simulink model "realtime_simu_franka_fr3"  (R2022b)
settings: Solver=FixedStepDiscrete  StartTime=0.0  StopTime=inf  FixedStep=0.001  RelTol=1e-3
PreLoadFcn:
  | set_param(gcs, 'RTWSystemTargetFile', 'franka_emika_panda.tlc');
  | 
  | demos_common_configs();
  | collision_behavior = ones(1,52)*100;
InitFcn:
  | parameters_franka_fr3;
values from neighbouring files (symbols this model uses):
  q_init = [0, -pi/4, 0, -3 * pi/4, 0, pi/2, pi/4]'    [parameters.m]    (also in parameters_franka_fr3.m)
undefined symbols (not defined in the file or in its folder): init_bus_param, MPC12, param_EKF, param_global, param_robot, param_savgol, param_traj, param_vis, v7_kin_int_planner
libraries: franka_simulink_library x5, dspstat3 x2
settings Model: SimulationMode=external  ExtModeTrigDuration=10000  Creator=vasi_ko  LastModifiedBy=rslstudent
settings SolverCC: AlgebraicLoopSolver=TrustRegion
settings DataIOCC: LimitDataPoints=on  SaveFormat=Array  ReturnWorkspaceOutputs=off
settings OptimizationCC: EnhancedBackFolding=on  OptimizeBlockOrder=speed  DifferentSizesBufferReuse=on  OptimizationCustomize=off
settings DebuggingCC: SolverPrmCheckMsg=warning  ParameterTunabilityLossMsg=error  UnconnectedInputMsg=warning  UnconnectedOutputMsg=warning  UnconnectedLineMsg=warning  SFUnexpectedBacktrackingDiag=warning  SFNoUnconditionalDefaultTransitionDiag=warning  SFExecutionAtInitializationDiag=none  SFMachineParentedDataDiag=warning  ArithmeticOperatorsInVariantConditions=warning
settings HardwareCC: ProdBitPerLong=64  ProdHWDeviceType=Intel->x86-64 (Linux 64)
settings ModelReferenceCC: UpdateModelReferenceTargets=IfOutOfDate  EnableRefExpFcnMdlSchedulingChecks=on  PropagateSignalLabelsOutOfModel=off
settings SFSimCC: SimUseLocalCustomCode=off  MATLABDynamicMemAlloc=off  CustomCodeUndefinedFunction=UseInterfaceOnly  SimTargetLang=C++
settings RTWCC: SystemTargetFile=franka_emika_panda.tlc  RTWUseLocalCustomCode=off  Toolchain=Franka Simulink | gmake (64-bit linux)  BuildConfiguration=Faster Runs  TargetLang=C++
settings CodeAppCC: OperatorAnnotations=on
settings STFCustomTargetCC: TargetLangStandard=C99 (ISO)  ModelReferenceCompliant=off  CombineOutputUpdateFcns=on  MatFileLogging=on  UseToolchainInfoCompliant=on  SystemTargetFile=franka_emika_panda.tlc
settings GRTTargetCC: ModelReferenceCompliant=off  ParMdlRefBuildCompliant=off  CompOptLevelCompliant=off  ConcurrentExecutionCompliant=off  CPPClassGenCompliant=off  ExtModeStaticAlloc=on  ExtModeTransport=1  ExtModeMexFile=ext_xcp  ExtModeIntrfLevel=Level2 - Open
settings ConfigComp: CovMetricSettings=dw  CovSaveCumulativeToWorkspaceVar=on  CovSaveSingleToWorkspaceVar=on  CovExternalEMLEnable=off  CovSFcnEnable=off

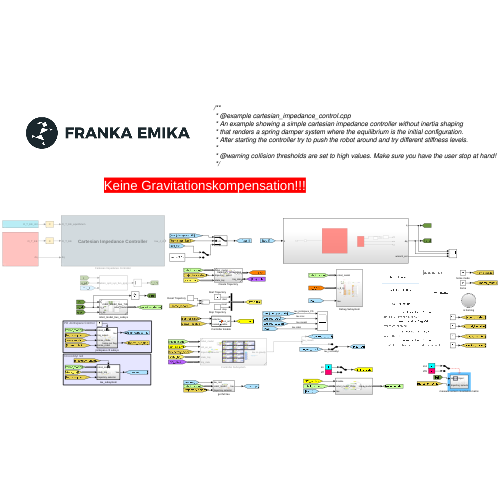
[thumbnail: Simulink's stored preview of the top-level diagram]
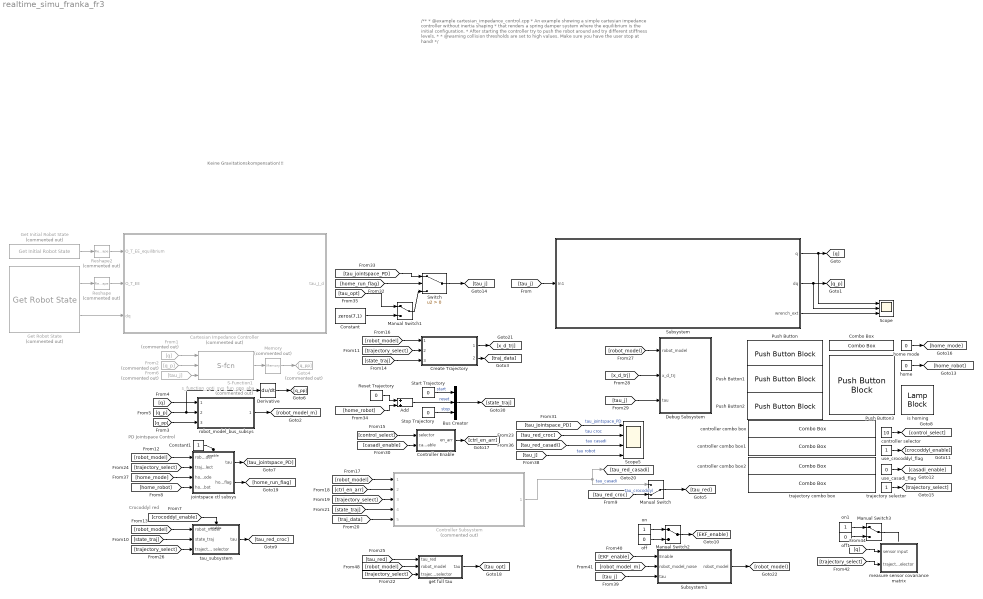
== system realtime_simu_franka_fr3 ==
  note: Crocoddyl red
  note: PD Jointspace Control
  note: Keine Gravitationskompensation!!!
  note: /**
      |  * @example cartesian_impedance_control.cpp
      |  * An example showing a simple cartesian impedance controller without inertia shaping
      |  * that renders a spring damper system where the equilibrium is the initial configuration.
      |  * After starting the controller try to push the robot around and try different stiffness levels.
      |  *
      |  * @warning collision thresholds are set to high values. Make sure you have the user stop at hand!
      |  */
  Add : Sum
  Bus Creator : BusCreator  Inputs=3  OutDataTypeStr=Bus: state_traj_bus
      settings: InheritFromInputs=off
  Cartesian Impedance Controller : Subsystem  Commented=on
      mask Display:
      | disp('{\bf\fontsize{18}Cartesian Impedance Controller}', 'texmode','on');
      | 
      | block_icon('Controller')
      | 
      | port_label('output',1,'tau_J_d');
      | 
      | port_label('input',1,'O_T_EE_equilibrium');
      | port_label('input',2,'O_T_EE');
      | port_label('input',3,'dq');
  Combo Box : ComboBox  LabelPosition=Hide  SelectedLabel=Home init pose
      settings: Values={{'Home init pose', 'Trajectory init pose'}, [0 1]}
  Constant : Constant  Value=zeros(7,1)
  Constant1 : Constant
  Controller Enable : MATLAB Function  TreatAsAtomicUnit=on
  Controller Subsystem : Subsystem  Commented=on  ReferencedSubsystem=controller_ref_subsys
  Create Trajectory : Subsystem  ReferencedSubsystem=trajectory_generation_ref_subsys_7dof
  Debug Subsystem : Subsystem
  Derivative : Derivative
  From1 : From  Commented=on  GotoTag=q
  From2 : From  Commented=on  GotoTag=q_p
  From6 : From  Commented=on  GotoTag=tau_j
  Get Initial Robot State : franka_simulink_library/Get Initial Robot State  Commented=on  robot_ip=robot_ip  signals_requested='O_T_EE'
      settings: SourceProductName=Franka Emika Simulink Support Package
  Get Robot State : franka_simulink_library/Get Robot State  Commented=on  robot_ip=robot_ip  signals_requested='O_T_EE dq'
      settings: SourceProductName=Franka Emika Simulink Support Package
  Goto4 : Goto  Commented=on  GotoTag=q_pp
  Manual Switch : ManualSwitch  CurrentSetting=0
  Manual Switch1 : ManualSwitch
  Manual Switch2 : ManualSwitch
  Manual Switch3 : ManualSwitch
  Memory : Memory  Commented=on  InitialCondition=zeros(7,1)
  Push Button : PushButtonBlock  ButtonText=Start Trajectory  OffValue=0.000000
  Push Button1 : PushButtonBlock  ButtonText=Reset Trajectory  OffValue=0.000000
  Push Button2 : PushButtonBlock  ButtonText=Stop Trajectory  OffValue=0.000000
  Push Button3 : PushButtonBlock  ButtonText=HOME ROBOT  OffValue=0.000000
  Reset Trajectory : Constant  Value=0
  Reshape : Reshape  Commented=on  OutputDimensionality=Customize  OutputDimensions=[4,4]
  Reshape2 : Reshape  Commented=on  OutputDimensionality=Customize  OutputDimensions=[4,4]
  S-Function1 : S-Function  Commented=on  FunctionName=s_function_opti_sys_fun_qpp_aba  SFunctionModules='sys_fun_qpp_aba'  SFunctionDeploymentMode=off  EnableBusSupport=off
  Scope : Scope  NumInputPorts=3
  Scope5 : Scope  NumInputPorts=4
  Start Trajectory : Constant  Value=0
  Stop Trajectory : Constant  Value=0
  Subsystem : Subsystem
  Subsystem1 : Subsystem
  Switch : Switch  Criteria=u2 > Threshold  SaturateOnIntegerOverflow=off  InputSameDT=off
  controller combo box : ComboBox  SelectedLabel=MPC12 (v7_kin_int_planner)
      settings: Values={{'Cartesian CT Control', 'Cartesian PD+ Control', 'MPC01', 'MPC6 (v3_quat)', 'MPC7 (v3_rpy)', 'MPC8 (v4_kin_int)', 'MPC9 (v4_kin_int_refsys)', 'MPC10 (v5_kin_dev)', 'MPC11 (v6_kin_int_pathfollow)', 'MPC12 (v7_kin_int_planner)', 'MPC13 (v8_kin_dev_planner)'}, [1 2 3 4 5 6 7 8 9 10 11]}
  controller combo box1 : ComboBox  SelectedLabel=Croccodyl Enabled
      settings: Values={{'Croccodyl Enabled', 'Croccodyl Disabled'}, [1 0]}
  controller combo box2 : ComboBox  SelectedLabel=Casadi Disabled
      settings: Values={{'Casadi Enabled', 'Casadi Disabled'}, [1 0]}
  controller selector : Constant  Value=10  OutDataTypeStr=uint32  SampleTime=-1
  get full tau : Subsystem
  home : Constant  Value=0
  home mode : Constant  Value=0
  is homing : LampBlock  LabelPosition=Hide
  jointspace ctl subsys : Subsystem
  measure sensor covariance matrix : Subsystem
  off : Constant  Value=0
  off1 : Constant  Value=0
  on : Constant
  on1 : Constant
  robot_model_bus_subsys : Subsystem  ReferencedSubsystem=robot_model_bus_7dof_ref_subsys
  tau_subsystem : Subsystem
  trajectory combo box : ComboBox  SelectedLabel=1: Singularity stretched arm out, Polynomial, Workspace
      settings: Values={{'1: Singularity stretched arm out, Polynomial, Workspace', '2: Singularity stretched arm in, Polynomial, Workspace', '3: Wrist singularity 1, Polynomial, Workspace', '4: Wrist singularity 1, Polynomial, Jointspace', '5: Shoulder - Wrist singularity 1, Polynomial, Workspace'}, [1 2 3 4 5]}
  trajectory selector : Constant  OutDataTypeStr=uint32  SampleTime=-1
  use_casadi_flag : Constant  Value=0
  use_crocoddyl_flag : Constant
  wires:
  Reshape2/1 -> Cartesian Impedance Controller/1(O_T_EE_equilibrium)
  Get Initial Robot State/1 -> Reshape2/1
  Subsystem/1(q) -> Scope/1, [q]
  Subsystem/2(dq) -> Scope/2, [q_p]
  Get Robot State/2 -> Cartesian Impedance Controller/3(dq)
  Reshape/1 -> Cartesian Impedance Controller/2(O_T_EE)
  Get Robot State/1 -> Reshape/1
  Subsystem/3(wrench_ext) -> Scope/3
  [tau_jointspace_PD] -> Scope5/1  "tau_jointspace_PD"
  [tau_j] -> Subsystem/1(In1)
  [q] -> robot_model_bus_subsys/1
  robot_model_bus_subsys/1 -> [robot_model_m]
  [q_p] -> Derivative/1, robot_model_bus_subsys/2
  [q_pp] -> robot_model_bus_subsys/3
  From6/1 -> S-Function1/3
  From1/1 -> S-Function1/1
  From2/1 -> S-Function1/2
  Start Trajectory/1 -> Bus Creator/1  "start"
  Stop Trajectory/1 -> Bus Creator/3  "stop"
  Bus Creator/1 -> [state_traj]
  Constant1/1 -> jointspace ctl subsys/Enable
  [robot_model] -> jointspace ctl subsys/1(robot_model)
  jointspace ctl subsys/1(tau) -> [tau_jointspace_PD]
  [robot_model] -> tau_subsystem/1(robot_model)
  tau_subsystem/1(tau) -> [tau_red_croc]
  [control_select] -> Controller Enable/1(selector)
  Controller Enable/1(en_arr) -> [ctrl_en_arr]
  [robot_model] -> Controller Subsystem/1
  [ctrl_en_arr] -> Controller Subsystem/2
  [trajectory_select] -> Controller Subsystem/3
  [tau_red_croc] -> Manual Switch/2  "tau_crocoddyl"
  [state_traj] -> tau_subsystem/2(state_traj)
  [trajectory_select] -> get full tau/3(trajectory selector)
  [robot_model] -> get full tau/2(robot_model)
  [tau_red] -> get full tau/1(tau_red)
  get full tau/1(tau) -> [tau_opt]
  Manual Switch/1 -> [tau_red]
  Controller Subsystem/1 -> Manual Switch/1, [tau_red_casadi]  "tau_casadi"
  [trajectory_select] -> tau_subsystem/3(trajectory selector)
  [tau_red_croc] -> Scope5/2  "tau croc"
  [crocoddyl_enable] -> tau_subsystem/Enable
  [robot_model] -> Debug Subsystem/1(robot_model)
  [x_d_trj] -> Debug Subsystem/2(x_d_trj)
  [tau_j] -> Debug Subsystem/3(tau)
  Derivative/1 -> [q_pp]
  use_crocoddyl_flag/1 -> [crocoddyl_enable]
  use_casadi_flag/1 -> [casadi_enable]
  [casadi_enable] -> Controller Enable/2(casadi_enable)
  S-Function1/1 -> Memory/1
  Memory/1 -> Goto4/1
  home/1 -> [home_robot]
  [home_robot] -> jointspace ctl subsys/4(home_robot)
  jointspace ctl subsys/2(home run flag) -> [home_run_flag]
  [home_run_flag] -> Switch/2
  [tau_jointspace_PD] -> Switch/1
  Reset Trajectory/1 -> Add/1
  Add/1 -> Bus Creator/2  "reset"
  [home_robot] -> Add/2
  [tau_red_casadi] -> Scope5/3  "tau casadi"
  Create Trajectory/2 -> [traj_data]
  [robot_model] -> Create Trajectory/1
  [trajectory_select] -> Create Trajectory/2
  Create Trajectory/1 -> [x_d_trj]
  [state_traj] -> Create Trajectory/3
  controller selector/1 -> [control_select]
  trajectory selector/1 -> [trajectory_select]
  home mode/1 -> [home_mode]
  [home_mode] -> jointspace ctl subsys/3(home_mode)
  [trajectory_select] -> jointspace ctl subsys/2(traj_select)
  [state_traj] -> Controller Subsystem/4
  [traj_data] -> Controller Subsystem/5
  [tau_j] -> Scope5/4  "tau robot"
  Constant/1 -> Manual Switch1/2
  [tau_opt] -> Manual Switch1/1
  Manual Switch1/1 -> Switch/3
  Switch/1 -> [tau_j]
  on/1 -> Manual Switch2/1
  Manual Switch2/1 -> [EKF_enable]
  [robot_model_m] -> Subsystem1/2(robot_model_noise)
  [tau_j] -> Subsystem1/3(tau)
  off/1 -> Manual Switch2/2
  [EKF_enable] -> Subsystem1/1(Enable)
  Subsystem1/1(robot_model) -> [robot_model]
  [q] -> measure sensor covariance matrix/1(sensor input)
  off1/1 -> Manual Switch3/2
  on1/1 -> Manual Switch3/1
  Manual Switch3/1 -> ?
  [trajectory_select] -> measure sensor covariance matrix/2(trajectory selector)

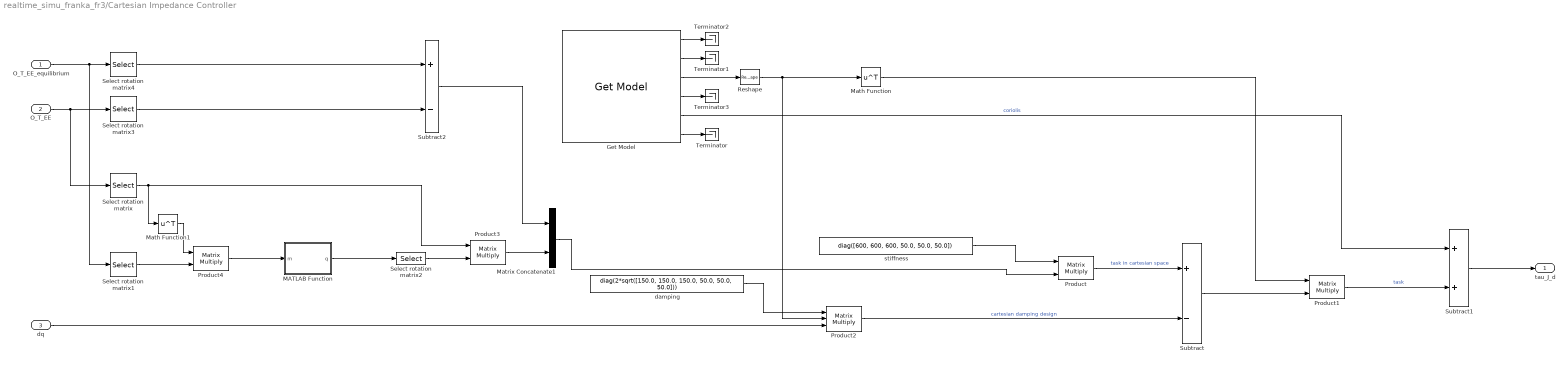
== system realtime_simu_franka_fr3/Cartesian Impedance Controller ==
  O_T_EE_equilibrium : Inport
  O_T_EE : Inport  Port=2
  dq : Inport  Port=3
  Get Model : franka_simulink_library/Get Model  robot_ip=robot_ip
      settings: SourceProductName=Franka Emika Simulink Support Package
  MATLAB Function : MATLAB Function  TreatAsAtomicUnit=on
  Math Function : Math  Operator=transpose  SignedPower=on
  Math Function1 : Math  Operator=transpose  SignedPower=on
  Matrix Concatenate1 : Concatenate
  Product{,1,3..4} (4 alike) : Product  Multiplication=Matrix(*)
  Product2 : Product  Inputs=3  Multiplication=Matrix(*)
  Reshape : Reshape  OutputDimensionality=Customize  OutputDimensions=[6,7]
  Select rotation matrix : Selector  NumberOfDimensions=2  InputPortWidth=3  IndexOptions=Index vector (dialog),Index vector (dialog)  Indices=[1,2,3],[1 2 3]  OutputSizes=1
  Select rotation matrix1 : Selector  NumberOfDimensions=2  InputPortWidth=3  IndexOptions=Index vector (dialog),Index vector (dialog)  Indices=[1,2,3],[1 2 3]  OutputSizes=1
  Select rotation matrix2 : Selector  InputPortWidth=4  IndexOptions=Index vector (dialog)  Indices=[2,3,4]  OutputSizes=1
  Select rotation matrix3 : Selector  NumberOfDimensions=2  InputPortWidth=3  IndexOptions=Index vector (dialog),Index vector (dialog)  Indices=[1,2,3],[4]  OutputSizes=1
  Select rotation matrix4 : Selector  NumberOfDimensions=2  InputPortWidth=3  IndexOptions=Index vector (dialog),Index vector (dialog)  Indices=[1,2,3],[4]  OutputSizes=1
  Subtract : Sum  Inputs=+-
  Subtract1 : Sum
  Subtract2 : Sum  Inputs=+-
  Terminator{,1..3} (4 alike) : Terminator
  damping : Constant  Value=diag(2*sqrt([150.0, 150.0, 150.0, 50.0, 50.0, 50.0]))  VectorParams1D=off
  stiffness : Constant  Value=diag([600, 600, 600, 50.0, 50.0, 50.0])  VectorParams1D=off
  tau_J_d : Outport  VectorParamsAs1DForOutWhenUnconnected=off
  wires:
  Get Model/6 -> Terminator/1
  Get Model/2 -> Terminator1/1
  Get Model/1 -> Terminator2/1
  Get Model/4 -> Terminator3/1
  Get Model/3 -> Reshape/1
  Reshape/1 -> Product2/2, Math Function/1
  stiffness/1 -> Product/1
  Math Function/1 -> Product1/1
  Product/1 -> Subtract/1  "task in cartesian space"
  Product2/1 -> Subtract/2  "cartesian damping design"
  Get Model/5 -> Subtract1/1  "coriolis"
  dq/1 -> Product2/3
  damping/1 -> Product2/1
  Subtract1/1 -> tau_J_d/1
  Product1/1 -> Subtract1/2  "task"
  O_T_EE/1 -> Select rotation matrix3/1, Select rotation matrix/1
  O_T_EE_equilibrium/1 -> Select rotation matrix4/1, Select rotation matrix1/1
  Select rotation matrix4/1 -> Subtract2/1
  Select rotation matrix3/1 -> Subtract2/2
  Subtract2/1 -> Matrix Concatenate1/1
  MATLAB Function/1(q) -> Select rotation matrix2/1
  Product4/1 -> MATLAB Function/1(m)
  Subtract/1 -> Product1/2
  Select rotation matrix2/1 -> Product3/2
  Matrix Concatenate1/1 -> Product/2
  Select rotation matrix/1 -> Math Function1/1, Product3/1
  Product3/1 -> Matrix Concatenate1/2
  Select rotation matrix1/1 -> Product4/2
  Math Function1/1 -> Product4/1

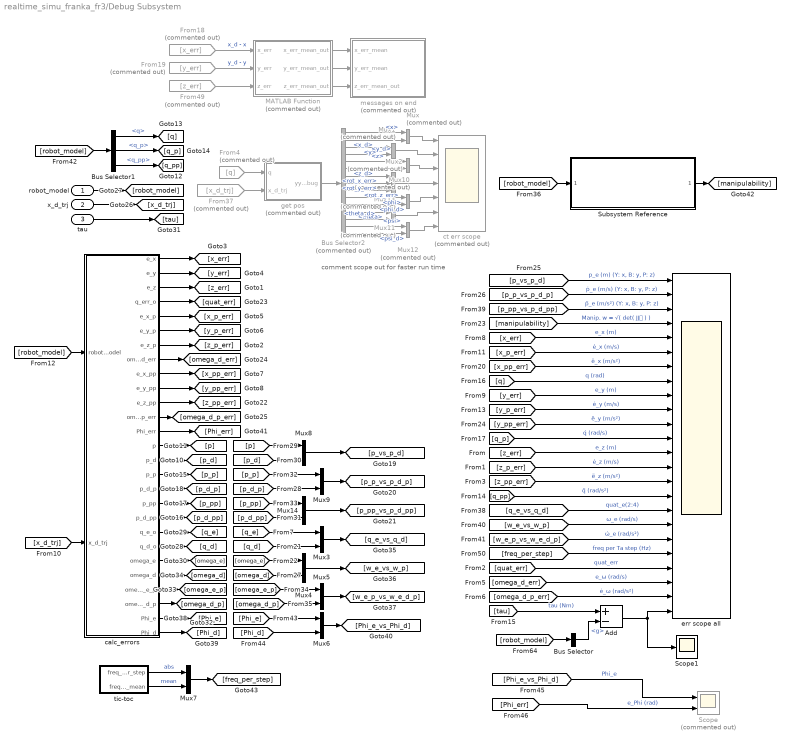
== system realtime_simu_franka_fr3/Debug Subsystem ==
  note: comment scope out for faster run time
  robot_model : Inport
  x_d_trj : Inport  Port=2
  tau : Inport  Port=3
  Add : Sum  Inputs=+-
  Bus Selector : BusSelector  OutputSignals=g
  Bus Selector1 : BusSelector  OutputSignals=q,q_p,q_pp
  Bus Selector2 : BusSelector  Commented=on  OutputSignals=x,x_d,y,y_d,z,z_d,rot_x_err,rot_y_err,rot_z_err,phi,phi_d,theta,theta_d,psi,psi_d
  From18 : From  Commented=on  GotoTag=x_err
  From19 : From  Commented=on  GotoTag=y_err
  From37 : From  Commented=on  GotoTag=x_d_trj
  From4 : From  Commented=on  GotoTag=q
  From49 : From  Commented=on  GotoTag=z_err
  MATLAB Function : MATLAB Function  Commented=on  TreatAsAtomicUnit=on
  Mux{,1..2,10..12} (6 alike) : Mux  Commented=on  Inputs=2
  Mux13 : Mux  Commented=on  Inputs=3
  Mux{3..9,14} (8 alike) : Mux  Inputs=2
  Scope : Scope  Commented=on  NumInputPorts=2
  Scope1 : Scope
  Subsystem Reference : Subsystem  ReferencedSubsystem=manipulability_and_collinearity
  calc_errors : MATLAB Function  TreatAsAtomicUnit=on
  ct err scope : Scope  Commented=on  NumInputPorts=7
  err scope all : Scope  NumInputPorts=24
  get pos : MATLAB Function  Commented=on  TreatAsAtomicUnit=on  SystemSampleTime=param_global.Ta
  messages on end : Subsystem  Commented=on
  tic-toc : Subsystem
  wires:
  Bus Selector1/1 -> [q]  "<q>"
  Bus Selector1/2 -> [q_p]  "<q_p>"
  Bus Selector1/3 -> [q_pp]  "<q_pp>"
  From4/1 -> get pos/1(q)
  x_d_trj/1 -> [x_d_trj]
  robot_model/1 -> [robot_model]
  tau/1 -> [tau]
  From37/1 -> get pos/2(x_d_trj)
  get pos/1(yy_debug) -> Bus Selector2/1
  Mux/1 -> ct err scope/1
  Mux1/1 -> ct err scope/2
  Mux2/1 -> ct err scope/3
  Mux10/1 -> ct err scope/5
  Mux11/1 -> ct err scope/6
  Mux12/1 -> ct err scope/7
  Mux13/1 -> ct err scope/4
  Bus Selector2/1 -> Mux/1  "<x>"
  Bus Selector2/2 -> Mux/2  "<x_d>"
  Bus Selector2/3 -> Mux1/1  "<y>"
  Bus Selector2/4 -> Mux1/2  "<y_d>"
  Bus Selector2/5 -> Mux2/1  "<z>"
  Bus Selector2/6 -> Mux2/2  "<z_d>"
  Bus Selector2/7 -> Mux13/1  "<rot_x_err>"
  Bus Selector2/8 -> Mux13/2  "<rot_y_err>"
  Bus Selector2/9 -> Mux13/3  "<rot_z_err>"
  Bus Selector2/10 -> Mux10/1  "<phi>"
  Bus Selector2/11 -> Mux10/2  "<phi_d>"
  Bus Selector2/12 -> Mux11/1  "<theta>"
  Bus Selector2/13 -> Mux11/2  "<theta_d>"
  Bus Selector2/14 -> Mux12/1  "<psi>"
  Bus Selector2/15 -> Mux12/2  "<psi_d>"
  From18/1 -> MATLAB Function/1(x_err)  "x_d - x"
  From19/1 -> MATLAB Function/2(y_err)  "y_d - y"
  MATLAB Function/2(y_err_mean_out) -> messages on end/2(y_err_mean)
  MATLAB Function/1(x_err_mean_out) -> messages on end/1(x_err_mean)
  [robot_model] -> calc_errors/1(robot_model)
  [x_d_trj] -> calc_errors/2(x_d_trj)
  calc_errors/1(e_x) -> [x_err]
  calc_errors/2(e_y) -> [y_err]
  calc_errors/5(e_x_p) -> [x_p_err]
  calc_errors/6(e_y_p) -> [y_p_err]
  calc_errors/9(e_x_pp) -> [x_pp_err]
  calc_errors/10(e_y_pp) -> [y_pp_err]
  [manipulability] -> err scope all/4  "Manip. w = √( det( JJ⸆ ) )"
  [x_err] -> err scope all/5  "e_x (m)"
  [y_err] -> err scope all/9  "e_y (m)"
  [x_p_err] -> err scope all/6  "ė_x (m/s)"
  [y_p_err] -> err scope all/10  "ė_y (m/s)"
  [x_pp_err] -> err scope all/7  "ё_x (m/s²)"
  [y_pp_err] -> err scope all/11  "ё_y (m/s²)"
  [q] -> err scope all/8  "q (rad)"
  [q_p] -> err scope all/12  "q̇ (rad/s)"
  [q_pp] -> err scope all/16  "q̈ (rad/s²)"
  [p_d_p] -> Mux9/2
  [p_p] -> Mux9/1
  [p_d] -> Mux8/2
  [p] -> Mux8/1
  [p_pp] -> Mux14/1
  [p_d_pp] -> Mux14/2
  [p_p_vs_p_d_p] -> err scope all/2  "ṗ_e (m/s) (Y: x, B: y, P: z)"
  [p_vs_p_d] -> err scope all/1  "p_e (m) (Y: x, B: y, P: z)"
  [p_pp_vs_p_d_pp] -> err scope all/3  "p̈_e (m/s²) (Y: x, B: y, P: z)"
  Mux8/1 -> [p_vs_p_d]
  Mux9/1 -> [p_p_vs_p_d_p]
  Mux14/1 -> [p_pp_vs_p_d_pp]
  calc_errors/14(p) -> [p]
  calc_errors/15(p_d) -> [p_d]
  calc_errors/16(p_p) -> [p_p]
  calc_errors/17(p_d_p) -> [p_d_p]
  calc_errors/18(p_pp) -> [p_pp]
  calc_errors/19(p_d_pp) -> [p_d_pp]
  calc_errors/3(e_z) -> [z_err]
  calc_errors/7(e_z_p) -> [z_p_err]
  calc_errors/11(e_z_pp) -> [z_pp_err]
  [z_err] -> err scope all/13  "e_z (m)"
  [z_p_err] -> err scope all/14  "ė_z (m/s)"
  [z_pp_err] -> err scope all/15  "ё_z (m/s²)"
  calc_errors/4(q_err_o) -> [quat_err]
  calc_errors/12(omega_d_p_err) -> [omega_d_p_err]
  calc_errors/8(omega_d_err) -> [omega_d_err]
  [quat_err] -> err scope all/21  "quat_err"
  [omega_d_err] -> err scope all/22  "e_ω (rad/s)"
  [omega_d_p_err] -> err scope all/23  "ė_ω (rad/s²)"
  calc_errors/20(q_e_o) -> [q_e]
  calc_errors/21(q_d_o) -> [q_d]
  calc_errors/22(omega_e) -> [omega_e]
  calc_errors/23(omega_d) -> [omega_d]
  calc_errors/24(omega_e_p) -> [omega_e_p]
  calc_errors/25(omega_d_p) -> [omega_d_p]
  [q_e] -> Mux3/1
  [q_d] -> Mux3/2
  [omega_e] -> Mux4/1
  [omega_d] -> Mux4/2
  [omega_e_p] -> Mux5/1
  [omega_d_p] -> Mux5/2
  Mux3/1 -> [q_e_vs_q_d]
  Mux4/1 -> [w_e_vs_w_p]
  Mux5/1 -> [w_e_p_vs_w_e_d_p]
  [q_e_vs_q_d] -> err scope all/17  "quat_e(2:4)"
  [w_e_vs_w_p] -> err scope all/18  "ω_e (rad/s)"
  [w_e_p_vs_w_e_d_p] -> err scope all/19  "ὠ_e (rad/s²)"
  calc_errors/26(Phi_e) -> [Phi_e]
  calc_errors/27(Phi_d) -> [Phi_d]
  [Phi_d] -> Mux6/2
  [Phi_e] -> Mux6/1
  Mux6/1 -> [Phi_e_vs_Phi_d]
  [Phi_e_vs_Phi_d] -> Scope/1  "Phi_e"
  calc_errors/13(Phi_err) -> [Phi_err]
  [Phi_err] -> Scope/2  "e_Phi (rad)"
  From49/1 -> MATLAB Function/3(z_err)
  MATLAB Function/3(z_err_mean_out) -> messages on end/3(z_err_mean_out)
  [freq_per_step] -> err scope all/20  "freq per Ta step (Hz)"
  Subsystem Reference/1 -> [manipulability]
  [robot_model] -> Subsystem Reference/1
  Mux7/1 -> [freq_per_step]
  tic-toc/1(freq_per_step) -> Mux7/1  "abs"
  tic-toc/2(freq_per_step_mean) -> Mux7/2  "mean"
  [robot_model] -> Bus Selector/1
  [tau] -> Add/1  "tau (Nm)"
  Add/1 -> err scope all/24, Scope1/1
  Bus Selector/1 -> Add/2  "<g>"
  [robot_model] -> Bus Selector1/1

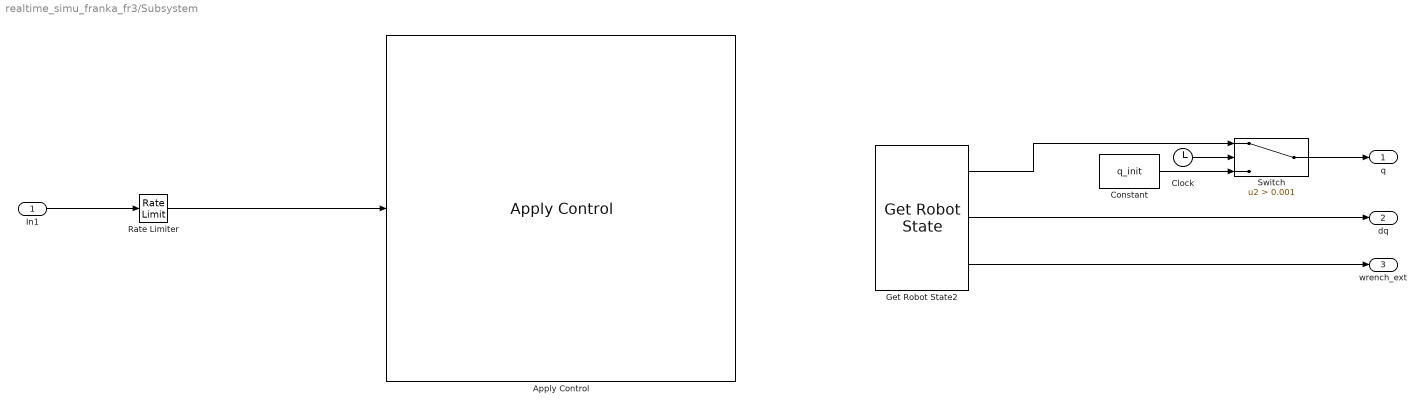
== system realtime_simu_franka_fr3/Subsystem ==
  In1 : Inport
  Apply Control : franka_simulink_library/Apply Control  robot_ip=robot_ip  gripper_attached=off  control_mode=Torque Control  controller_choice=Joint Impedance Controller  elbow_control=on  collision_thresholds=100*ones(1,52)  joint_impedance=joint_impedance  cartesian_impedance=cartesian_impedance  load_inertia=load_inertia  EE_T_K=EE_T_K  init_joint_configuration_req=on  init_joint_configuration=q_init'
      settings: SourceProductName=Franka Emika Simulink Support Package
  Clock : Clock
  Constant : Constant  Value=q_init
  Get Robot State2 : franka_simulink_library/Get Robot State  robot_ip=robot_ip  signals_requested='q dq O_F_ext_hat_K'
      settings: SourceProductName=Franka Emika Simulink Support Package
  Rate Limiter : RateLimiter  RisingSlewLimit=1000  FallingSlewLimit=-1000  SampleTimeMode=inherited
  Switch : Switch  Criteria=u2 > Threshold  Threshold=0.001  SaturateOnIntegerOverflow=off  InputSameDT=off
  q : Outport
  dq : Outport  Port=2
  wrench_ext : Outport  Port=3
  wires:
  Clock/1 -> Switch/2
  Constant/1 -> Switch/3
  Get Robot State2/3 -> wrench_ext/1
  Get Robot State2/2 -> dq/1
  In1/1 -> Rate Limiter/1
  Get Robot State2/1 -> Switch/1
  Switch/1 -> q/1
  Rate Limiter/1 -> Apply Control/1

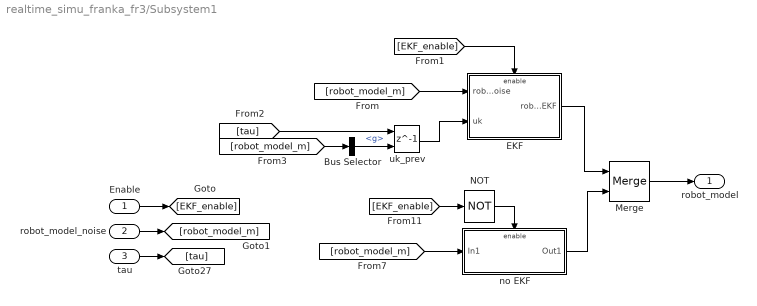
== system realtime_simu_franka_fr3/Subsystem1 ==
  Enable : Inport
  robot_model_noise : Inport  Port=2  OutDataTypeStr=Bus: robot_model
  tau : Inport  Port=3
  Bus Selector : BusSelector  OutputSignals=g
  EKF : Subsystem
  Merge : Merge
  NOT : Logic  Operator=NOT  IconShape=distinctive  AllPortsSameDT=off  OutDataTypeStr=boolean
  no EKF : Subsystem
  uk_prev : Delay  DelayLength=1  InitialConditionSource=Input port
      settings: InputPortMap=u0,p4
  robot_model : Outport  OutDataTypeStr=Bus: robot_model
  wires:
  [robot_model_m] -> no EKF/1(In1)
  no EKF/1(Out1) -> Merge/2
  uk_prev/1 -> EKF/2(uk)
  [EKF_enable] -> NOT/1
  Merge/1 -> robot_model/1
  Bus Selector/1 -> uk_prev/2  "<g>"
  [robot_model_m] -> EKF/1(robot_model_noise)
  EKF/1(robot_model_EKF) -> Merge/1
  NOT/1 -> no EKF/Enable
  [EKF_enable] -> EKF/Enable
  Enable/1 -> [EKF_enable]
  robot_model_noise/1 -> [robot_model_m]
  tau/1 -> [tau]
  [tau] -> uk_prev/1
  [robot_model_m] -> Bus Selector/1

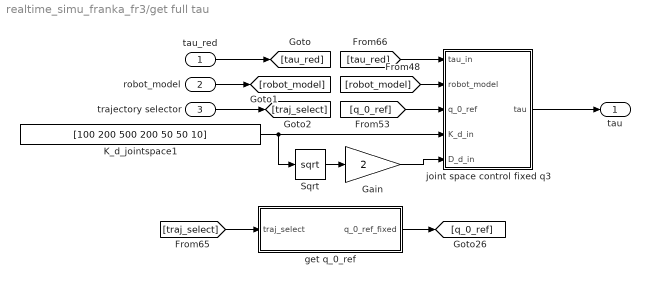
== system realtime_simu_franka_fr3/get full tau ==
  tau_red : Inport
  robot_model : Inport  Port=2
  trajectory selector : Inport  Port=3
  Gain : Gain  Gain=2
  K_d_jointspace1 : Constant  Value=[100 200 500 200 50 50 10]
  Sqrt : Sqrt
  get q_0_ref : MATLAB Function  TreatAsAtomicUnit=on
  joint space control fixed q3 : MATLAB Function  TreatAsAtomicUnit=on
  tau : Outport
  wires:
  [traj_select] -> get q_0_ref/1(traj_select)
  [q_0_ref] -> joint space control fixed q3/3(q_0_ref)
  get q_0_ref/1(q_0_ref_fixed) -> [q_0_ref]
  Sqrt/1 -> Gain/1
  joint space control fixed q3/1(tau) -> tau/1
  Gain/1 -> joint space control fixed q3/5(D_d_in)
  [tau_red] -> joint space control fixed q3/1(tau_in)
  tau_red/1 -> [tau_red]
  [robot_model] -> joint space control fixed q3/2(robot_model)
  robot_model/1 -> [robot_model]
  trajectory selector/1 -> [traj_select]
  K_d_jointspace1/1 -> Sqrt/1, joint space control fixed q3/4(K_d_in)

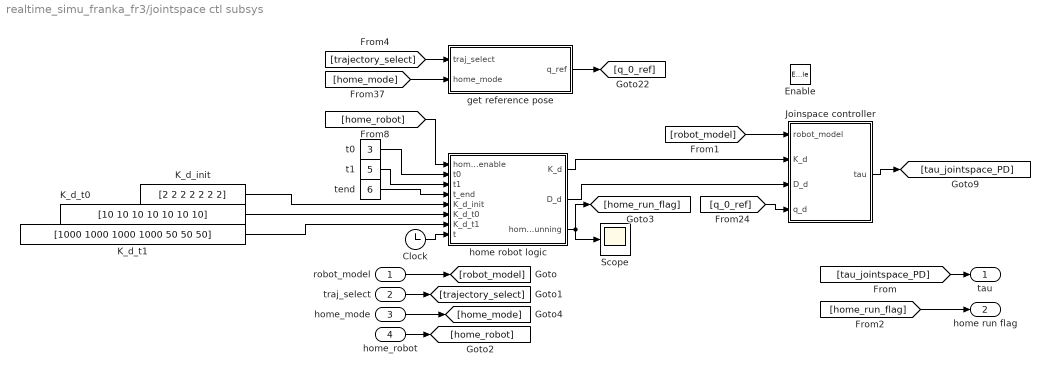
== system realtime_simu_franka_fr3/jointspace ctl subsys ==
  robot_model : Inport  OutDataTypeStr=Bus: robot_model
  traj_select : Inport  Port=2
  home_mode : Inport  Port=3
  home_robot : Inport  Port=4
  Enable : EnablePort
  Clock : Clock
  Joinspace controller : MATLAB Function  TreatAsAtomicUnit=on
  K_d_init : Constant  Value=[2 2 2 2 2 2 2]
  K_d_t0 : Constant  Value=[10 10 10 10 10 10 10]
  K_d_t1 : Constant  Value=[1000 1000 1000 1000 50 50 50]
  Scope : Scope
  get reference pose : MATLAB Function  TreatAsAtomicUnit=on
  home robot logic : MATLAB Function  TreatAsAtomicUnit=on
  t0 : Constant  Value=3
  t1 : Constant  Value=5
  tend : Constant  Value=6
  tau : Outport
  home run flag : Outport  Port=2
  wires:
  [tau_jointspace_PD] -> tau/1
  robot_model/1 -> [robot_model]
  [q_0_ref] -> Joinspace controller/4(q_d)
  Joinspace controller/1(tau) -> [tau_jointspace_PD]
  [robot_model] -> Joinspace controller/1(robot_model)
  home robot logic/1(K_d) -> Joinspace controller/2(K_d)
  home_robot/1 -> [home_robot]
  [home_robot] -> home robot logic/1(home_robot_enable)
  Clock/1 -> home robot logic/8(t)
  home robot logic/3(home_running) -> [home_run_flag], Scope/1
  [home_run_flag] -> home run flag/1
  t0/1 -> home robot logic/2(t0)
  t1/1 -> home robot logic/3(t1)
  tend/1 -> home robot logic/4(t_end)
  home robot logic/2(D_d) -> Joinspace controller/3(D_d)
  get reference pose/1(q_ref) -> [q_0_ref]
  traj_select/1 -> [trajectory_select]
  [trajectory_select] -> get reference pose/1(traj_select)
  [home_mode] -> get reference pose/2(home_mode)
  home_mode/1 -> [home_mode]
  K_d_init/1 -> home robot logic/5(K_d_init)
  K_d_t0/1 -> home robot logic/6(K_d_t0)
  K_d_t1/1 -> home robot logic/7(K_d_t1)

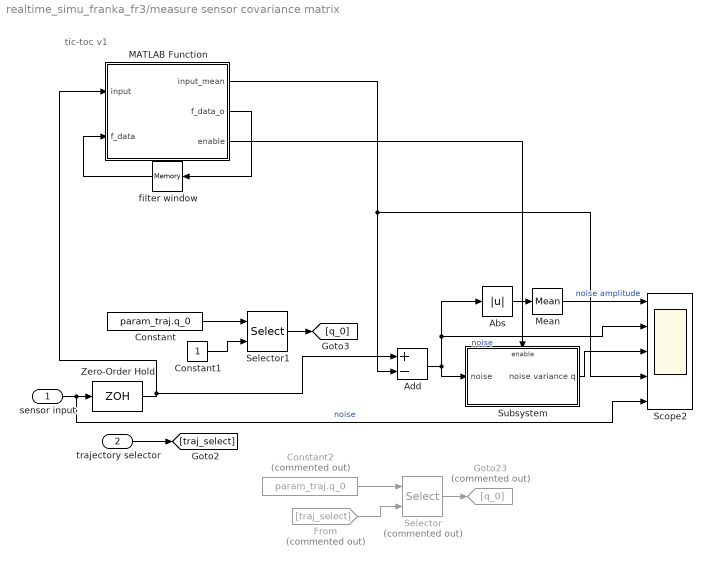
== system realtime_simu_franka_fr3/measure sensor covariance matrix ==
  note: tic-toc v1
  sensor input : Inport
  trajectory selector : Inport  Port=2
  Abs : Abs  SaturateOnIntegerOverflow=off
  Add : Sum  Inputs=+-
  Constant : Constant  Value=param_traj.q_0
  Constant1 : Constant
  Constant2 : Constant  Commented=on  Value=param_traj.q_0
  From : From  Commented=on  GotoTag=traj_select
  Goto23 : Goto  Commented=on  GotoTag=q_0
  MATLAB Function : MATLAB Function  TreatAsAtomicUnit=on
  Mean : dspstat3/Mean  run=on  InputProcessing=Columns as channels (frame based)  reset_popup=None  directionMode=Each column  dimension=1  roiEnable=off  roiType=Rectangles  roiPortion=Entire ROI  roiOutput=Individual statistics for each ROI  roiFlag=off  roundingMode=Floor  overflowMode=off  outputDataTypeStr=Inherit: Same as accumulator  outputMin=[]  outputMax=[]  outputLastDataTypeStr=Inherit: Same as accumulator
  Scope2 : Scope  NumInputPorts=5
  Selector : Selector  Commented=on  NumberOfDimensions=2  InputPortWidth=3  IndexOptions=Index vector (dialog),Index vector (port)  Indices=1:param_robot.n_DOF,1  OutputSizes=1,1
  Selector1 : Selector  NumberOfDimensions=2  InputPortWidth=3  IndexOptions=Index vector (dialog),Index vector (port)  Indices=1:param_robot.n_DOF,1  OutputSizes=1,1
  Subsystem : Subsystem
  Zero-Order Hold : ZeroOrderHold  SampleTime=-1
  filter window : Memory  InitialCondition=zeros(param_savgol.N_n, param_robot.n_DOF)
  wires:
  From/1 -> Selector/2
  Selector/1 -> Goto23/1
  Constant2/1 -> Selector/1
  trajectory selector/1 -> [traj_select]
  MATLAB Function/1(input_mean) -> Scope2/4, Add/2
  filter window/1 -> MATLAB Function/2(f_data)
  MATLAB Function/2(f_data_o) -> filter window/1
  Abs/1 -> Mean/1
  Selector1/1 -> [q_0]
  Constant1/1 -> Selector1/2
  Add/1 -> Subsystem/1(noise), Abs/1, Scope2/2  "noise"
  Mean/1 -> Scope2/1  "noise amplitude"
  Constant/1 -> Selector1/1
  sensor input/1 -> Scope2/5, Zero-Order Hold/1  "noise"
  Zero-Order Hold/1 -> Add/1, MATLAB Function/1(input)
  MATLAB Function/3(enable) -> Subsystem/Enable
  Subsystem/1(noise variance q) -> Scope2/3

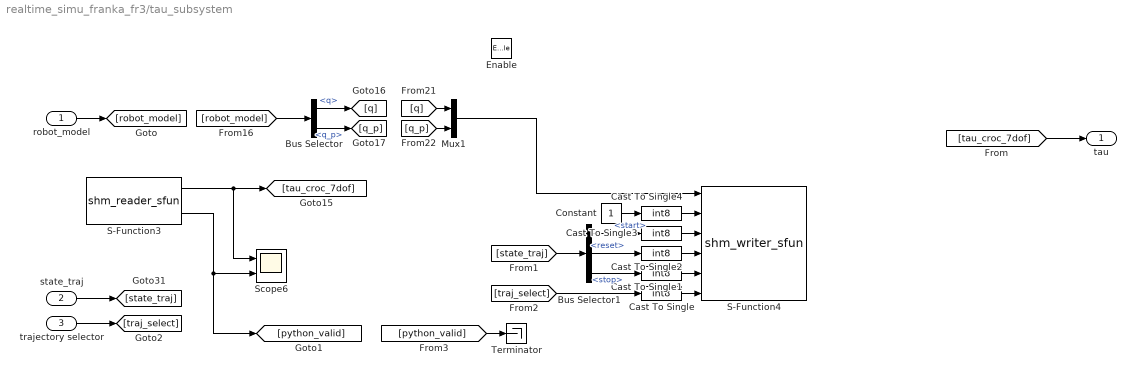
== system realtime_simu_franka_fr3/tau_subsystem ==
  robot_model : Inport  OutDataTypeStr=Bus: robot_model
  state_traj : Inport  Port=2  OutDataTypeStr=Bus: state_traj_bus
  trajectory selector : Inport  Port=3
  Enable : EnablePort
  Bus Selector : BusSelector  OutputSignals=q,q_p
  Bus Selector1 : BusSelector  OutputSignals=start,reset,stop
  Cast To Single{,1..4} (5 alike) : DataTypeConversion  OutDataTypeStr=int8  SaturateOnIntegerOverflow=off  RndMeth=Floor
  Constant : Constant
  Mux1 : Mux  Inputs=2
  S-Function3 : S-Function  FunctionName=shm_reader_sfun  Parameters='data_from_python', 'data_from_python_valid'  SFunctionDeploymentMode=off  EnableBusSupport=off
  S-Function4 : S-Function  FunctionName=shm_writer_sfun  Parameters='data_from_simulink', 'data_from_simulink_valid', 'data_from_simulink_start', 'data_from_simulink_reset', 'data_from_simulink_stop', 'data_from_simulink_traj_switch'  SFunctionDeploymentMode=off  EnableBusSupport=off
  Scope6 : Scope  NumInputPorts=2
  Terminator : Terminator
  tau : Outport
  wires:
  Bus Selector/2 -> [q_p]  "<q_p>"
  Mux1/1 -> S-Function4/1
  S-Function3/1 -> Scope6/1, [tau_croc_7dof]
  [robot_model] -> Bus Selector/1
  [q] -> Mux1/1
  S-Function3/2 -> [python_valid], Scope6/2
  Bus Selector/1 -> [q]  "<q>"
  [q_p] -> Mux1/2
  robot_model/1 -> [robot_model]
  state_traj/1 -> [state_traj]
  [state_traj] -> Bus Selector1/1
  Bus Selector1/3 -> Cast To Single1/1  "<stop>"
  trajectory selector/1 -> [traj_select]
  [traj_select] -> Cast To Single/1
  [python_valid] -> Terminator/1
  Cast To Single/1 -> S-Function4/6
  Cast To Single1/1 -> S-Function4/5
  Bus Selector1/2 -> Cast To Single2/1  "<reset>"
  Cast To Single2/1 -> S-Function4/4
  Cast To Single3/1 -> S-Function4/3
  Bus Selector1/1 -> Cast To Single3/1  "<start>"
  Cast To Single4/1 -> S-Function4/2
  Constant/1 -> Cast To Single4/1
  [tau_croc_7dof] -> tau/1

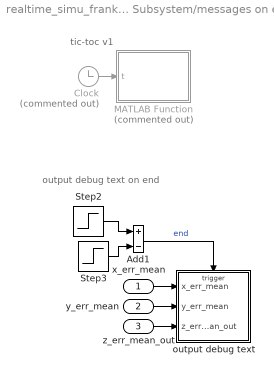
== system realtime_simu_franka_fr3/Debug Subsystem/messages on end ==
  note: tic-toc v1
  note: output debug text on end
  x_err_mean : Inport
  y_err_mean : Inport  Port=2
  z_err_mean_out : Inport  Port=3
  Add1 : Sum  Inputs=+-
  Clock : Clock  Commented=on
  MATLAB Function : MATLAB Function  Commented=on  TreatAsAtomicUnit=on
  Step2 : Step  Time=param_vis.T-param_global.Ta  SampleTime=param_global.Ta
  Step3 : Step  Time=param_vis.T  SampleTime=param_global.Ta
  output debug text : Subsystem  TreatAsAtomicUnit=on
  wires:
  Clock/1 -> MATLAB Function/1(t)
  Add1/1 -> output debug text/Trigger  "end"
  Step3/1 -> Add1/2
  Step2/1 -> Add1/1
  y_err_mean/1 -> output debug text/2(y_err_mean)
  x_err_mean/1 -> output debug text/1(x_err_mean)
  z_err_mean_out/1 -> output debug text/3(z_err_mean_out)

== system realtime_simu_franka_fr3/Debug Subsystem/tic-toc ==
  note: tic-toc v1
  MATLAB Function : MATLAB Function  TreatAsAtomicUnit=on
  filter window : Memory  InitialCondition=zeros(param_savgol.N, 1)
  freq_per_step : Outport
  freq_per_step_mean : Outport  Port=2
  wires:
  MATLAB Function/1(freq_per_step) -> freq_per_step/1
  filter window/1 -> MATLAB Function/1(f_data)
  MATLAB Function/2(freq_per_step_mean) -> freq_per_step_mean/1
  MATLAB Function/3(f_data_o) -> filter window/1

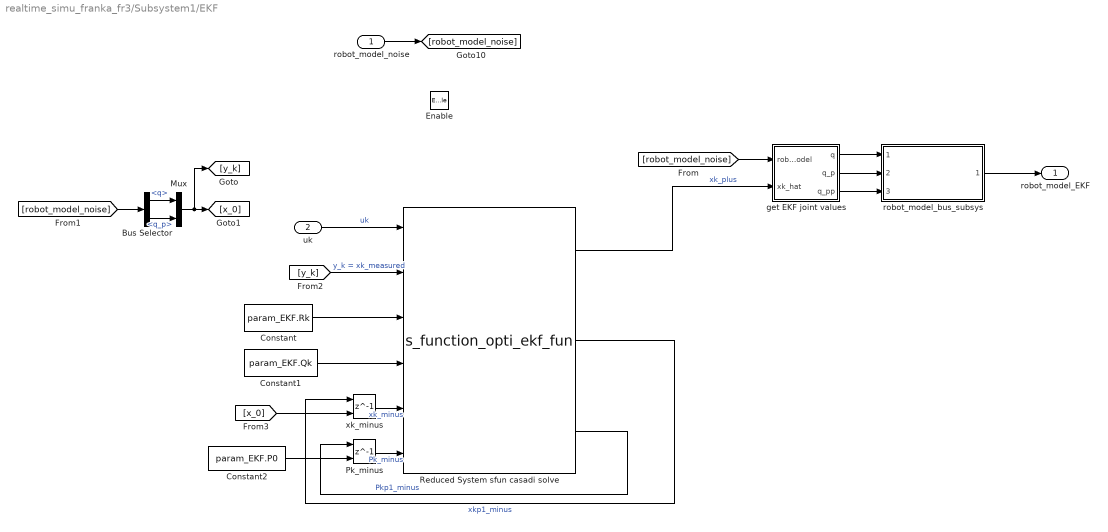
== system realtime_simu_franka_fr3/Subsystem1/EKF ==
  robot_model_noise : Inport  OutDataTypeStr=Bus: robot_model
  uk : Inport  Port=2
  Enable : EnablePort
  Bus Selector : BusSelector  OutputSignals=q,q_p
  Constant : Constant  Value=param_EKF.Rk
  Constant1 : Constant  Value=param_EKF.Qk
  Constant2 : Constant  Value=param_EKF.P0
  Mux : Mux  Inputs=2
  Pk_minus : Delay  DelayLength=1  InitialConditionSource=Input port
      settings: InputPortMap=u0,p4
  Reduced System sfun casadi solve : S-Function  FunctionName=s_function_opti_ekf_fun  SFunctionModules='ekf_fun'  SFunctionDeploymentMode=off  EnableBusSupport=off
  get EKF joint values : MATLAB Function  TreatAsAtomicUnit=on
  robot_model_bus_subsys : Subsystem  ReferencedSubsystem=robot_model_bus_7dof_ref_subsys
  xk_minus : Delay  DelayLength=1  InitialConditionSource=Input port
      settings: InputPortMap=u0,p4
  robot_model_EKF : Outport  OutDataTypeStr=Bus: robot_model
  wires:
  uk/1 -> Reduced System sfun casadi solve/1  "uk"
  Constant1/1 -> Reduced System sfun casadi solve/4
  Constant/1 -> Reduced System sfun casadi solve/3
  xk_minus/1 -> Reduced System sfun casadi solve/5  "xk_minus"
  Pk_minus/1 -> Reduced System sfun casadi solve/6  "Pk_minus"
  Reduced System sfun casadi solve/3 -> Pk_minus/1  "Pkp1_minus"
  Reduced System sfun casadi solve/2 -> xk_minus/1  "xkp1_minus"
  robot_model_noise/1 -> [robot_model_noise]
  [robot_model_noise] -> Bus Selector/1
  Reduced System sfun casadi solve/1 -> get EKF joint values/2(xk_hat)  "xk_plus"
  [robot_model_noise] -> get EKF joint values/1(robot_model)
  [y_k] -> Reduced System sfun casadi solve/2  "y_k = xk_measured"
  [x_0] -> xk_minus/2
  get EKF joint values/3(q_pp) -> robot_model_bus_subsys/3
  get EKF joint values/2(q_p) -> robot_model_bus_subsys/2
  get EKF joint values/1(q) -> robot_model_bus_subsys/1
  robot_model_bus_subsys/1 -> robot_model_EKF/1
  Constant2/1 -> Pk_minus/2
  Bus Selector/1 -> Mux/1  "<q>"
  Bus Selector/2 -> Mux/2  "<q_p>"
  Mux/1 -> [y_k], [x_0]

== system realtime_simu_franka_fr3/Subsystem1/no EKF ==
  In1 : Inport
  Enable : EnablePort
  Out1 : Outport
  wires:
  In1/1 -> Out1/1

== system realtime_simu_franka_fr3/measure sensor covariance matrix/Subsystem ==
  noise : Inport
  Enable : EnablePort
  Variance : dspstat3/Variance  run=on  InputProcessing=Columns as channels (frame based)  reset_popup=None  directionMode=Each row  dimension=1  roiEnable=off  roiType=Rectangles  roiPortion=Entire ROI  roiOutput=Individual statistics for each ROI  roiFlag=off  roundingMode=Floor  overflowMode=off
  noise variance q : Outport
  wires:
  noise/1 -> Variance/1
  Variance/1 -> noise variance q/1  "noise variance q"

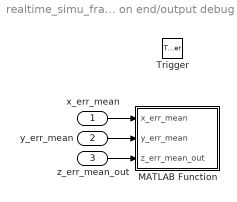
== system realtime_simu_franka_fr3/Debug Subsystem/messages on end/output debug text ==
  x_err_mean : Inport
  y_err_mean : Inport  Port=2
  z_err_mean_out : Inport  Port=3
  Trigger : TriggerPort  VariantControl=(inherit)
  MATLAB Function : MATLAB Function  TreatAsAtomicUnit=on
  wires:
  y_err_mean/1 -> MATLAB Function/2(y_err_mean)
  x_err_mean/1 -> MATLAB Function/1(x_err_mean)
  z_err_mean_out/1 -> MATLAB Function/3(z_err_mean_out)

== matlab function realtime_simu_franka_fr3/Debug Subsystem/get pos ==
  settings: updateMethod=DISCRETE  sampleTime=param_global.Ta
  data: q input; yy_debug output Bus: yy_debug_bus; param_robot parameter; x_d_trj input Bus: x_d; init_bus_param parameter
function yy_debug  = fcn(q, param_robot, x_d_trj, init_bus_param)

yy_debug = init_bus_param.init_yy_debug_bus;

H = hom_transform_endeffector(q, param_robot);
y_t_W_E = H(1:3,4);
y_t_W_E_d = x_d_trj.p_d;

R_W_E = H(1:3,1:3);
ori_t_W_E = rotm2eul(R_W_E, 'XYZ');
ori_t_W_E_d = rotm2eul(quaternion2rotation(x_d_trj.q_d), 'XYZ');

yy_debug.x =  y_t_W_E(1);
yy_debug.x_d = y_t_W_E_d(1);

yy_debug.y =  y_t_W_E(2);
yy_debug.y_d = y_t_W_E_d(2);

yy_debug.z =  y_t_W_E(3);
yy_debug.z_d = y_t_W_E_d(3);

yy_debug.phi = ori_t_W_E(1);
yy_debug.phi_d = ori_t_W_E_d(1);

yy_debug.theta = ori_t_W_E(2);
yy_debug.theta_d = ori_t_W_E_d(2);

yy_debug.psi = ori_t_W_E(3);
yy_debug.psi_d = ori_t_W_E_d(3);

quat_err = quat_mult(rotation2quaternion(R_W_E), quat_inv(x_d_trj.q_d));
yy_debug.rot_x_err = quat_err(2);
yy_debug.rot_y_err = quat_err(3);
yy_debug.rot_z_err = quat_err(4);

== matlab function realtime_simu_franka_fr3/Debug Subsystem/tic-toc/MATLAB Function ==
  settings: updateMethod=DISCRETE  sampleTime=param_global.Ta
  data: freq_per_step output; f_data input; freq_per_step_mean output; param_savgol parameter; f_data_o output
function [freq_per_step, freq_per_step_mean, f_data_o] = fcn(f_data, param_savgol)

persistent cnt;
persistent time_start

if(isempty(time_start))
    tic;
    cnt = 0;
    time_start = 0;
end

if(cnt > 1)
    time_end = toc;
    freq_per_step = 1/(time_end - time_start);
    freq_per_step_mean = param_savgol.bT * f_data;
    time_start = time_end;
else
    freq_per_step = 0;
    freq_per_step_mean = 0;
end

if(cnt < param_savgol.N)
    cnt = cnt + 1;
    f_data(cnt:end) = mean([f_data; freq_per_step]);
end

f_data_o = [freq_per_step; f_data(1:end-1, 1)];
%disp(['Simulink execution time: ', sprintf('%f', time_per_step), ' s']);

== matlab function realtime_simu_franka_fr3/jointspace ctl subsys/home robot logic ==
  data: K_d output; D_d output; home_robot_enable input; t0 input; t1 input; t_end input; K_d_init input; K_d_t0 input; K_d_t1 input; home_running output; t input
function [K_d, D_d, home_running]= fcn(home_robot_enable, t0, t1, t_end, K_d_init, K_d_t0, K_d_t1, t)

persistent enabled;
persistent t_start;

if(isempty(enabled))
    enabled = 0;
    t_start = t;
end

if(home_robot_enable == 1)
    enabled = 1;
    t_start = t;
end

if(t-t_start < t0)
    frac = (t - t_start) / (t0);
    K_d = K_d_init + frac * (K_d_t0 - K_d_init);
elseif(t-t_start < t1)
    frac = (t - t_start - t0) / (t1);
    K_d = K_d_init + frac * (K_d_t1 - K_d_t0);
else
    K_d = K_d_t1;
end

D_d = sqrt(2*K_d);

if(t-t_start > t_end)
    enabled = 0;
end

home_running = enabled;

== matlab function realtime_simu_franka_fr3/Controller Enable ==
  settings: sampleTime=param_global.Ta
  data: en_arr output; selector input uint32; casadi_enable input
function en_arr  = fcn(selector, casadi_enable)
    % Wichtig: selector \in [1,max(selector)]
    % Es wird ein bool array ausgegeben, welches nur den index 1 setzt, der
    % mit selector übereinstimmt. Achtung: Size von "en_arr" muss
    % entsprechend der Ausgänge unter "Edit Data" manuell angegeben werden.
    % Beispiel: 4 Inputs, max(selector)=4, Size = [1 4]
    % z. B. selector = 2
    % 1:4 == selector liefert [0 1 0 0]
    en_arr = casadi_enable*(1:11 == selector)';
end

== matlab function realtime_simu_franka_fr3/Debug Subsystem/messages on end/MATLAB Function ==
  settings: updateMethod=DISCRETE  sampleTime=param_global.Ta
  data: t input; param_vis parameter
function fcn(t, param_vis)

if(t==0)
    tic;
end

if(t==param_vis.T)
    toc;
end

== matlab function realtime_simu_franka_fr3/Subsystem1/EKF/get EKF joint values ==
  data: robot_model input Bus: robot_model; q output; xk_hat input; q_p output; q_pp output; param_robot parameter
function [q, q_p, q_pp] = fcn(robot_model, xk_hat, param_robot)

n_DOF = param_robot.n_DOF;

q = xk_hat(1:n_DOF);
q_p = xk_hat(n_DOF+1:2*n_DOF);
q_pp = robot_model.q_pp;

== matlab function realtime_simu_franka_fr3/Debug Subsystem/messages on end/output debug text/MATLAB Function ==
  settings: updateMethod=DISCRETE
  data: x_err_mean input; y_err_mean input; z_err_mean_out input
function fcn(x_err_mean, y_err_mean, z_err_mean_out)
    disp(['mean x_err = ', sprintf('%.6e', x_err_mean),     ' m']);
    disp(['mean y_err = ', sprintf('%.6e', y_err_mean),     ' m']);
    disp(['mean y_err = ', sprintf('%.6e', z_err_mean_out), ' m']);
end

== matlab function realtime_simu_franka_fr3/get full tau/get q_0_ref ==
  data: q_0_ref_fixed output; traj_select input; param_traj parameter
function q_0_ref_fixed = fcn(traj_select, param_traj)

q_0_ref_fixed = param_traj.q_0(:, traj_select);

== matlab function realtime_simu_franka_fr3/measure sensor covariance matrix/MATLAB Function ==
  settings: updateMethod=DISCRETE  sampleTime=param_global.Ta
  data: input input; f_data input; input_mean output; param_savgol parameter; f_data_o output; enable output
function [input_mean, f_data_o, enable] = fcn(input, f_data, param_savgol)

persistent cnt;

if(isempty(cnt))
    cnt = 0;
end

if(cnt < param_savgol.N_n+3000)
    cnt = cnt + 1;
    enable = 0;
else
    enable = 1;
end

input_mean = (param_savgol.bT_n * f_data)';

f_data_o = [input'; f_data(1:end-1, :)];

== matlab function realtime_simu_franka_fr3/Debug Subsystem/MATLAB Function ==
  data: x_err_mean_out output; x_err input; y_err input; y_err_mean_out output; z_err input; z_err_mean_out output
function [x_err_mean_out, y_err_mean_out, z_err_mean_out] = fcn(x_err, y_err, z_err)

persistent cnt;
persistent x_err_mean;
persistent y_err_mean;
persistent z_err_mean;

if(isempty(cnt))
    cnt = 1;
    x_err_mean = 0;
    y_err_mean = 0;
    z_err_mean = 0;
end
% m1 =  a          = (0*m0+a)/1
% m2 = (a+b)/2     = (1*m1+b)/2
% m3 = (a+b+c)/3   = (2*m2+c)/3
% m4 = (a+b+c+d)/4 = (3*m3+d)/4
% ...
% mi = ((i-1)*m_{i-1})/i; 
x_err_mean = ((cnt-1)*x_err_mean + x_err)/cnt;
y_err_mean = ((cnt-1)*y_err_mean + y_err)/cnt;
z_err_mean = ((cnt-1)*z_err_mean + z_err)/cnt;

x_err_mean_out = x_err_mean;
y_err_mean_out = y_err_mean;
z_err_mean_out = z_err_mean;

cnt = cnt + 1;

%Die iterative Methode ist anfälliger für Rundungsfehler.
%Die iterative Methode kann bei sehr großen Datenmengen numerisch instabil
% werden

== matlab function realtime_simu_franka_fr3/get full tau/joint space control fixed q3 ==
  data: tau_in input; tau output; robot_model input Bus: robot_model; q_0_ref input; K_d_in input; D_d_in input; param_robot parameter
function tau = fcn(tau_in, robot_model, q_0_ref, K_d_in, D_d_in, param_robot)

%g = robot_model.g;
q = robot_model.q;
q_p = robot_model.q_p;

n_indices_fixed = param_robot.n_indices_fixed;

q_0_ref_fix = q_0_ref(n_indices_fixed);

q_fix = q(n_indices_fixed);
q_p_fix = q_p(n_indices_fixed);
%g_fix = g(n_indices_fixed); is ignored

D_d = diag(D_d_in(n_indices_fixed));
K_d = diag(K_d_in(n_indices_fixed));

tau_fix_q = -K_d * (q_fix - q_0_ref_fix) -D_d*q_p_fix;

tau_in(n_indices_fixed) = tau_in(n_indices_fixed) + tau_fix_q;
tau = tau_in;

== matlab function realtime_simu_franka_fr3/Cartesian Impedance Controller/MATLAB Function ==
  data: m input; q output
function q = rotm2quat(m)

m00 = m(1,1);
m01 = m(1,2);
m02 = m(1,3);

m10 = m(2,1);
m11 = m(2,2);
m12 = m(2,3);

m20 = m(3,1);
m21 = m(3,2);
m22 = m(3,3);

tr = m00 + m11 + m22;

if (tr > 0) 
  S = sqrt(tr+1.0) * 2; % S=4*qw 
  qw = 0.25 * S;
  qx = (m21 - m12) / S;
  qy = (m02 - m20) / S; 
  qz = (m10 - m01) / S; 
elseif ((m00 > m11) && (m00 > m22))
  S = sqrt(1.0 + m00 - m11 - m22) * 2;  %S=4*qx 
  qw = (m21 - m12) / S;
  qx = 0.25 * S;
  qy = (m01 + m10) / S; 
  qz = (m02 + m20) / S; 
elseif (m11 > m22) 
  S = sqrt(1.0 + m11 - m00 - m22) * 2; % S=4*qy
  qw = (m02 - m20) / S;
  qx = (m01 + m10) / S; 
  qy = 0.25 * S;
  qz = (m12 + m21) / S; 
else 
  S = sqrt(1.0 + m22 - m00 - m11) * 2; % S=4*qz
  qw = (m10 - m01) / S;
  qx = (m02 + m20) / S;
  qy = (m12 + m21) / S;
  qz = 0.25 * S;
end

q = [qw,qx,qy,qz]';

== matlab function realtime_simu_franka_fr3/jointspace ctl subsys/get reference pose ==
  data: traj_select input; q_ref output; home_mode input; param_traj parameter
function q_ref = fcn(traj_select, home_mode, param_traj)
if(home_mode == 0)
    q_ref = [0, -pi/4, 0, -3 * pi/4, 0, pi/2, pi/4]';
else
    q_ref = param_traj.q_0(:, traj_select);
end

== matlab function realtime_simu_franka_fr3/jointspace ctl subsys/Joinspace controller ==
  settings: updateMethod=DISCRETE  sampleTime=param_global.Ta
  data: tau output; robot_model input Bus: robot_model; K_d input; D_d input; q_d input
function tau  = fcn(robot_model, K_d, D_d, q_d)

q = robot_model.q;
q_p = robot_model.q_p;

e_q = q - q_d;
tau = -diag(D_d)*q_p -diag(K_d)*e_q;

== matlab function realtime_simu_franka_fr3/Debug Subsystem/calc_errors ==
  data: robot_model input Bus: robot_model; e_x output; e_y output; e_z output; q_err_o output; e_x_p output; e_y_p output; e_z_p output; omega_d_err output; e_x_pp output; e_y_pp output; e_z_pp output; omega_d_p_err output; Phi_err output; x_d_trj input Bus: x_d; p output; p_d output; p_p output; p_d_p output; p_pp output; p_d_pp output; q_e_o output; q_d_o output; omega_e output; omega_d output; omega_e_p output; omega_d_p output; Phi_e output; Phi_d output
function [e_x, e_y, e_z, q_err_o, e_x_p, e_y_p, e_z_p, omega_d_err, e_x_pp, e_y_pp, e_z_pp, omega_d_p_err, Phi_err, p, p_d, p_p, p_d_p, p_pp, p_d_pp, q_e_o, q_d_o, omega_e, omega_d, omega_e_p, omega_d_p, Phi_e, Phi_d] = fcn(robot_model, x_d_trj)

p_d    = x_d_trj.p_d;
p_d_p  = x_d_trj.p_d_p;
p_d_pp = x_d_trj.p_d_pp;

R_d = x_d_trj.R_d;

q_d = x_d_trj.q_d;
omega_d = x_d_trj.omega_d;
omega_d_p = x_d_trj.omega_d_p;

% Parameters
q    = robot_model.q;      % generalized coordinates
q_p  = robot_model.q_p;  % time derivative of generalized coordinates
q_pp = robot_model.q_pp;
H    = robot_model.H;
J    = robot_model.J;
J_p  = robot_model.J_p;

R = H(1:3,1:3);% desired Orientation as rotational matrix

%y_q_err = quat_mult(y_q_e, quat_inv(param_traj_data.q_d(1:4, cnt, traj_select)));
q_err = rotm2quat_v4(R*R_d');
%y_q_e = rotm2quat_v4(R);
q_e = quat_mult(q_d, q_err);

% Current Pose of Endeffector
y = [H(1:3,4); q_e];
y_p = J*q_p;
y_pp = J*q_pp + J_p*q_p;



p           = y(1:3);
p_p         = y_p(1:3);
p_pp        = y_pp(1:3);
Phi_e     = rotm2eul_v2(R);
%Phi_e_p   = [0; 0; 0]; % ?????? Phi_p = T * omega?
%Phi_e_pp  = [0; 0; 0]; % ??????
q_e           = y(4:7);
omega_e       = y_p(4:6);
omega_e_p     = y_pp(4:6);

p_err       = y(1:3) - p_d;
p_p_err     = y_p(1:3) - p_d_p;
p_pp_err    = y_pp(1:3) - p_d_pp;
omega_err   = y_p(4:6)  - omega_d;
omega_p_err = y_pp(4:6) - omega_d_p;








%p    = debug_data.p;
%p_p  = debug_data.p_p;
%p_pp = debug_data.p_pp;

%q_e = debug_data.q;
%omega_e = debug_data.omega;
%omega_e_p = debug_data.omega_p;


q_e_o = q_e(2:4);
q_d_o = q_d(2:4);

e_x    = p_d(1)    - p(1);
e_x_p  = p_d_p(1)  - p_p(1);
e_x_pp = p_d_pp(1) - p_pp(1);

e_y    = p_d(2)    - p(2);
e_y_p  = p_d_p(2)  - p_p(2);
e_y_pp = p_d_pp(2) - p_pp(2);

e_z    = p_d(3)    - p(3);
e_z_p  = p_d_p(3)  - p_p(3);
e_z_pp = p_d_pp(3) - p_pp(3);

%q_err_full = quat_mult(q_e, quat_inv(q_d));
%q_err = q_err_full(2:4);
q_err_o = q_err(2:4);
omega_d_err = omega_e-omega_d;
omega_d_p_err = omega_e_p-omega_d_p;

R_e = quaternion2rotation(q_e);

%Phi_e = debug_data.Phi;
Phi_d = x_d_trj.Phi_d;
Phi_err = rotm2rpy(R_e*R_d');
